simulink model "RC_Circuit"  (R2024b)
settings: Solver=VariableStepAuto  StartTime=0.0  StopTime=50  RelTol=1e-3
undefined symbols (not defined in the file): C, R
settings Model: Creator=omari  LastModifiedBy=omari

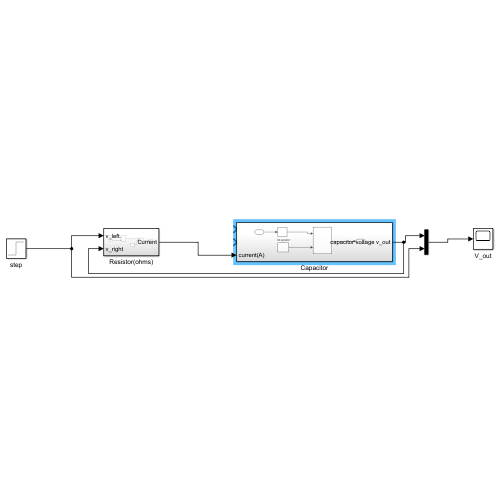
[thumbnail: Simulink's stored preview of the top-level diagram]
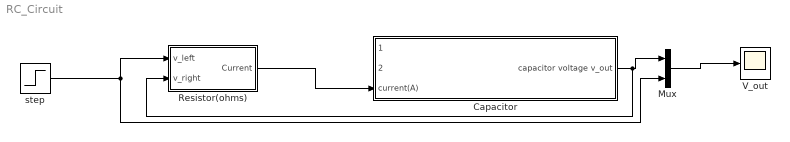
== system RC_Circuit ==
  Capacitor : Subsystem
  Mux : Mux  Inputs=2
  Resistor(ohms) : Subsystem
  V_out : Scope
  step : Step  SampleTime=0
  wires:
  step/1 -> Mux/2, Resistor(ohms)/1(v_left)
  Resistor(ohms)/1(Current) -> Capacitor/3(current(A))
  Mux/1 -> V_out/1
  Capacitor/1(capacitor voltage v_out) -> Resistor(ohms)/2(v_right), Mux/1

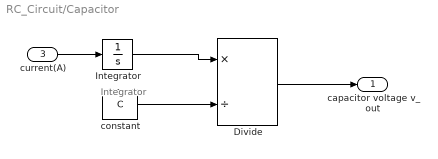
== system RC_Circuit/Capacitor ==
  note: Integrator
  current(A) : Inport  Port=3
  Divide : Product  Inputs=*/
  Integrator : Integrator
  constant : Constant  Value=C
  capacitor voltage v_out : Outport
  wires:
  Integrator/1 -> Divide/1
  current(A)/1 -> Integrator/1
  constant/1 -> Divide/2
  Divide/1 -> capacitor voltage v_out/1

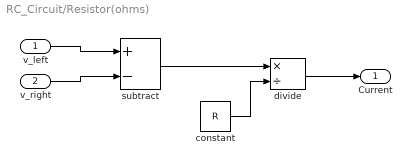
== system RC_Circuit/Resistor(ohms) ==
  v_left : Inport
  v_right : Inport  Port=2
  constant : Constant  Value=R
  divide : Product  Inputs=*/
  subtract : Sum  Inputs=+-
  Current : Outport
  wires:
  divide/1 -> Current/1
  v_left/1 -> subtract/1
  constant/1 -> divide/2
  v_right/1 -> subtract/2
  subtract/1 -> divide/1
